simulink model "Modele"  (R2018a)
settings: Solver=FixedStepAuto  StartTime=0.0  StopTime=1  FixedStep=0.000001  RelTol=1e-3
libraries: slctrlblks x1
settings Model: Creator=pt_ptsi  LastModifiedBy=pt_ptsi

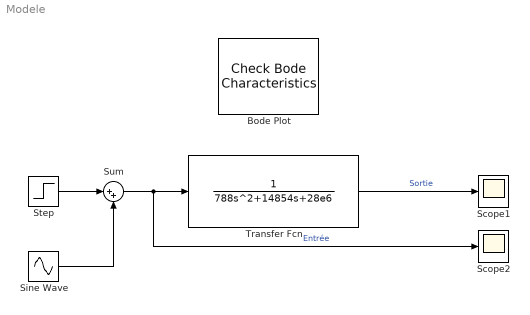
== system Modele ==
  Bode Plot : slctrlblks/Model Verification/Check Bode  Characteristics  InstantiateOnLoad=on  SaveOperatingPoints=off  LinearizationIOs={'/Sum', 1, 'in', 'on', '';'/Transfer Fcn', 1, 'out', 'on', ''}  LinearizeAt=SnapshotTimes  SnapshotTimes=[0]  TriggerType=rising  SampleTime=auto  RateConversionMethod=zoh  PreWarpFreq=10  UseExactDelayModel=off  UseFullBlockNameLabels=off  UseBusSignalLabels=off  enabled=on  stopWhenAssertionFail=off  export=off  ViewDlgPos=[1681 1 1680 974]  OpenViewOnLoad=off  LaunchViewOnOpen=off  FrequencyUnits=rad/s  MagnitudeUnits=dB  PhaseUnits=deg  TimeUnits=seconds  EnableUpperBound=off  UpperBoundFrequencies=[]  UpperBoundMagnitudes=[]  EnableLowerBound=off  LowerBoundFrequencies=[]  LowerBoundMagnitudes=[]
      settings: SourceProductName=Simulink Control Design
  Scope1 : Scope
  Scope2 : Scope
  Sine Wave : Sin  Amplitude=100  Frequency=3.5176e+04  SampleTime=0
  Step : Step  Time=0  After=1000  SampleTime=0
  Sum : Sum  Inputs=|++
  Transfer Fcn : TransferFcn  Denominator=[788 14854 28e6]
  wires:
  Step/1 -> Sum/1
  Sine Wave/1 -> Sum/2
  Sum/1 -> Scope2/1, Transfer Fcn/1  "Entrée"
  Transfer Fcn/1 -> Scope1/1  "Sortie"
